simulink model "cane"  (R2023b)
settings: Solver=FixedStepAuto  StartTime=0.0  StopTime=10.0  FixedStep=0.0001  RelTol=1e-3
settings Model: Creator=yuanluochen  LastModifiedBy=yuanluochen

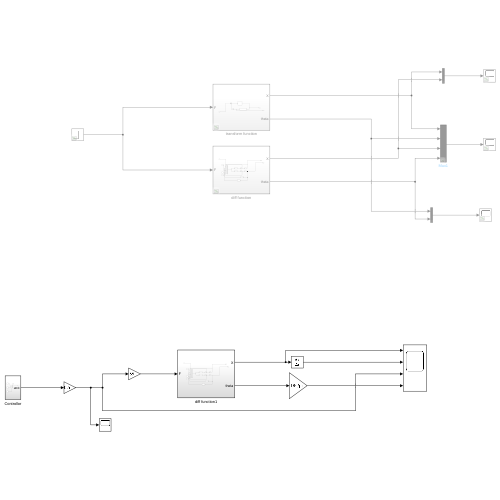
[thumbnail: Simulink's stored preview of the top-level diagram]
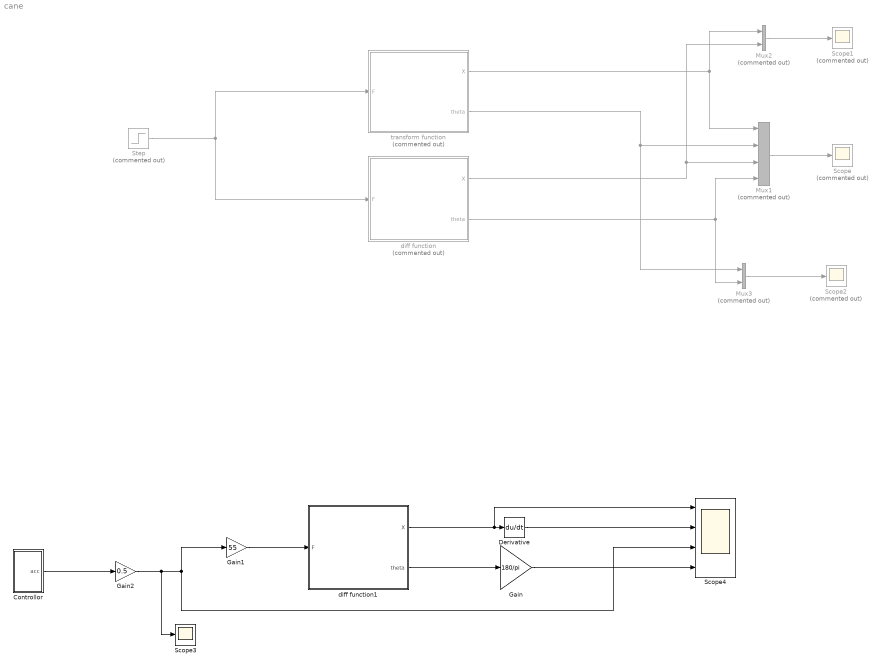
== system cane ==
  Controllor : Subsystem
  Derivative : Derivative
  Gain : Gain  Gain=180/pi
  Gain1 : Gain  Gain=55
  Gain2 : Gain  Gain=0.5
  Mux1 : Mux  Commented=on
  Mux2 : Mux  Commented=on  Inputs=2
  Mux3 : Mux  Commented=on  Inputs=2
  Scope : Scope  Commented=on
  Scope1 : Scope  Commented=on
  Scope2 : Scope  Commented=on
  Scope3 : Scope
  Scope4 : Scope  NumInputPorts=4
  Step : Step  Commented=on  Time=0  SampleTime=0
  diff function : Subsystem  Commented=on
  diff function1 : Subsystem
  transform function : Subsystem  Commented=on
  wires:
  Step/1 -> diff function/1(F), transform function/1(F)
  Mux1/1 -> Scope/1
  Mux2/1 -> Scope1/1
  Mux3/1 -> Scope2/1
  transform function/2(theta) -> Mux3/1, Mux1/2
  transform function/1(X) -> Mux2/1, Mux1/1
  diff function/2(theta) -> Mux3/2, Mux1/4
  diff function/1(X) -> Mux2/2, Mux1/3
  diff function1/1(X) -> Scope4/1, Derivative/1
  Derivative/1 -> Scope4/2
  diff function1/2(theta) -> Gain/1
  Gain/1 -> Scope4/4
  Gain1/1 -> diff function1/1(F)
  Gain2/1 -> Scope3/1, Scope4/3, Gain1/1
  Controllor/1(acc) -> Gain2/1

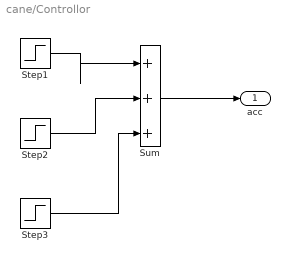
== system cane/Controllor ==
  Step1 : Step  Time=2  Before=1  After=0  SampleTime=0
  Step2 : Step  Time=5  After=-1  SampleTime=0
  Step3 : Step  Time=7  SampleTime=0
  Sum : Sum  Inputs=|+++
  acc : Outport
  wires:
  Step3/1 -> Sum/3
  Step1/1 -> Sum/1
  Step2/1 -> Sum/2
  Sum/1 -> acc/1

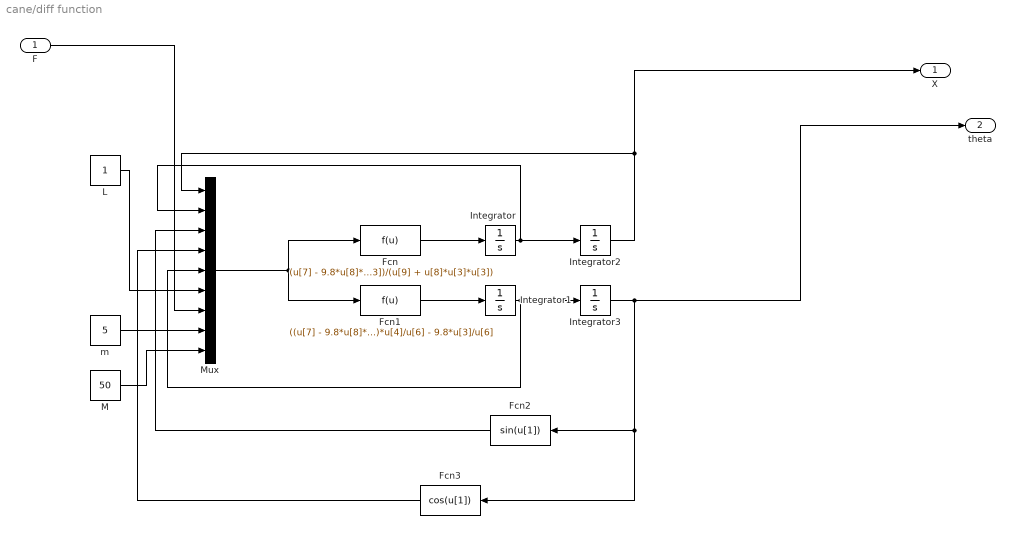
== system cane/diff function ==
  F : Inport
  Fcn : Fcn  Expr=(u[7] - 9.8*u[8]*u[3]*u[4] -u[8]*u[6]*u[5]*u[5]*u[3])/(u[9] + u[8]*u[3]*u[3])
  Fcn1 : Fcn  Expr=((u[7] - 9.8*u[8]*u[3]*u[4] -u[8]*u[6]*u[5]*u[5]*u[3])/(u[9] + u[8]*u[3]*u[3]))*u[4]/u[6] - 9.8*u[3]/u[6]
  Fcn2 : Fcn
  Fcn3 : Fcn  Expr=cos(u[1])
  Integrator{,1..3} (4 alike) : Integrator
  L : Constant
  M : Constant  Value=50
  Mux : Mux  Inputs=9
  m : Constant  Value=5
  X : Outport
  theta : Outport  Port=2
  wires:
  Fcn/1 -> Integrator/1
  Fcn2/1 -> Mux/3
  Fcn3/1 -> Mux/4
  Integrator1/1 -> Mux/5, Integrator3/1
  Mux/1 -> Fcn/1, Fcn1/1
  L/1 -> Mux/6
  M/1 -> Mux/9
  Fcn1/1 -> Integrator1/1
  m/1 -> Mux/8
  Integrator2/1 -> X/1, Mux/1
  Integrator3/1 -> theta/1, Fcn2/1, Fcn3/1
  Integrator/1 -> Mux/2, Integrator2/1
  F/1 -> Mux/7

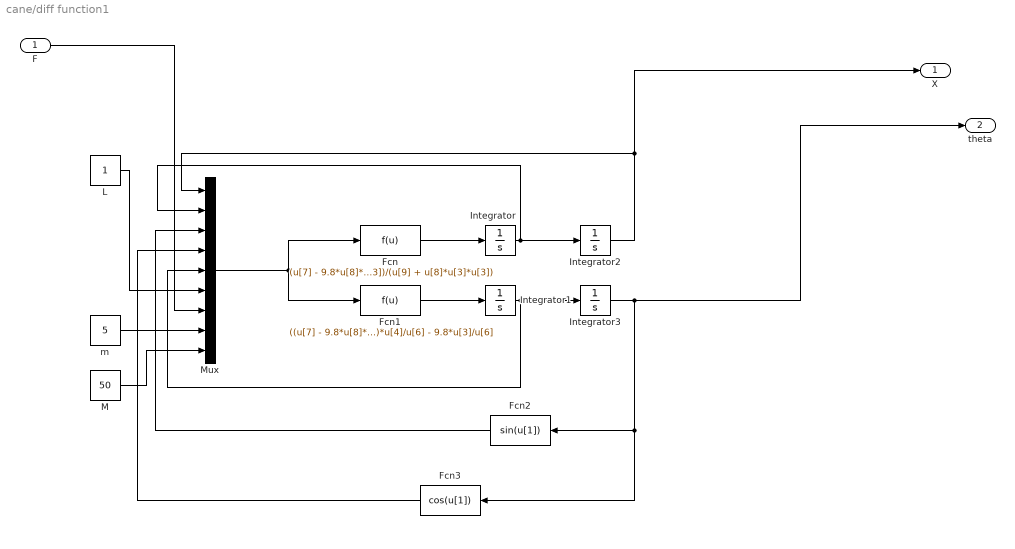
== system cane/diff function1 ==
  F : Inport
  Fcn : Fcn  Expr=(u[7] - 9.8*u[8]*u[3]*u[4] -u[8]*u[6]*u[5]*u[5]*u[3])/(u[9] + u[8]*u[3]*u[3])
  Fcn1 : Fcn  Expr=((u[7] - 9.8*u[8]*u[3]*u[4] -u[8]*u[6]*u[5]*u[5]*u[3])/(u[9] + u[8]*u[3]*u[3]))*u[4]/u[6] - 9.8*u[3]/u[6]
  Fcn2 : Fcn
  Fcn3 : Fcn  Expr=cos(u[1])
  Integrator{,1..3} (4 alike) : Integrator
  L : Constant
  M : Constant  Value=50
  Mux : Mux  Inputs=9
  m : Constant  Value=5
  X : Outport
  theta : Outport  Port=2
  wires:
  Fcn/1 -> Integrator/1
  Fcn2/1 -> Mux/3
  Fcn3/1 -> Mux/4
  Integrator1/1 -> Mux/5, Integrator3/1
  Mux/1 -> Fcn/1, Fcn1/1
  L/1 -> Mux/6
  M/1 -> Mux/9
  Fcn1/1 -> Integrator1/1
  m/1 -> Mux/8
  Integrator2/1 -> X/1, Mux/1
  Integrator3/1 -> theta/1, Fcn2/1, Fcn3/1
  Integrator/1 -> Mux/2, Integrator2/1
  F/1 -> Mux/7

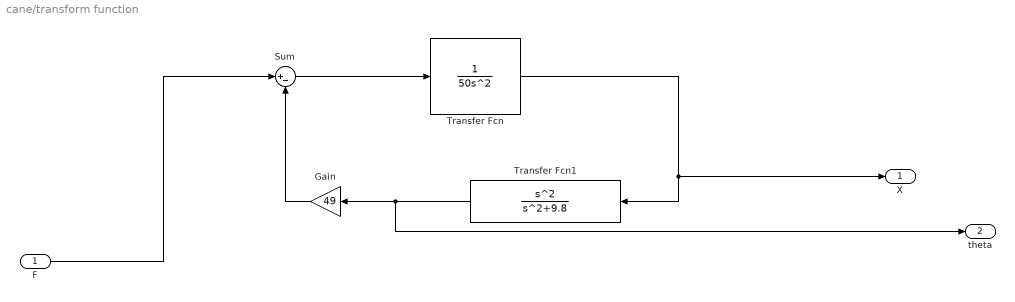
== system cane/transform function ==
  F : Inport
  Gain : Gain  Gain=49
  Sum : Sum  Inputs=|+-
  Transfer Fcn : TransferFcn  Denominator=[50 0 0]
  Transfer Fcn1 : TransferFcn  Numerator=[1 0 0]  Denominator=[1 0 9.8]
  X : Outport
  theta : Outport  Port=2
  wires:
  Sum/1 -> Transfer Fcn/1
  Gain/1 -> Sum/2
  Transfer Fcn/1 -> X/1, Transfer Fcn1/1
  F/1 -> Sum/1
  Transfer Fcn1/1 -> theta/1, Gain/1
